simulink model "adc_preproc_core"  (R2012b)
settings: Solver=VariableStepDiscrete  SolverMode=SingleTasking  StartTime=0.0  StopTime=40960  RelTol=1e-3
undefined symbols (not defined in the file or in its folder): A, B, fixpnt, PCIN, xlipgetpartsetting
libraries: xbsIndex_r4 x537, casper_library_sources x8, casper_library_misc x8, simulink x1
(part 6 of 9)

== system adc_preproc_core/adc_preproc_core/noise_gen0/noise5/wgn/u2n ==
  u : Inport
  Delay : xbsIndex_r4/Delay  rst=off  infoeditControl=Selection of Reset will increase slice count due to use of real FFs and instead of SRLs  en=off  latency=1  dbl_ovrd=off  reg_retiming=off  block_type=delay
  Delay1 : xbsIndex_r4/Delay  rst=off  infoeditControl=Selection of Reset will increase slice count due to use of real FFs and instead of SRLs  en=off  latency=1  dbl_ovrd=off  reg_retiming=off  block_type=delay
  Delay2 : xbsIndex_r4/Delay  rst=off  infoeditControl=Selection of Reset will increase slice count due to use of real FFs and instead of SRLs  en=off  latency=1  dbl_ovrd=off  reg_retiming=off  block_type=delay
  Gateway Out : xbsIndex_r4/Gateway Out  inherit_from_input=off  hdl_port=off  timing_constraint=None  locs_specified=off  LOCs={}  UseAsDAC=off  DACChannel='1'  block_type=gatewayout
      settings: infoedit="Gateway out block.  Converts Xilinx fixed point inputs into ouputs of type Simulink integer, double, or fixed point.<P><P>Hardware notes:  In hardware these blocks become top level output ports or are discarded, depending on how they are configured."  xl_area=[0 0 0 0 17 0 0]  block_version=10.1.3
  Gateway Out1 : xbsIndex_r4/Gateway Out  inherit_from_input=off  hdl_port=off  timing_constraint=None  locs_specified=off  LOCs={}  UseAsDAC=off  DACChannel='1'  block_type=gatewayout
      settings: infoedit="Gateway out block.  Converts Xilinx fixed point inputs into ouputs of type Simulink integer, double, or fixed point.<P><P>Hardware notes:  In hardware these blocks become top level output ports or are discarded, depending on how they are configured."  xl_area=[0 0 0 0 17 0 0]  block_version=10.1.3
  Scope : Scope  NumInputPorts=2
      settings: YMin=-5~-5  YMax=5~5
  bottom_11 : xbsIndex_r4/Slice  nbits=11  boolean_output=off  mode=Lower Bit Location + Width  bit1=0  base1=MSB of Input  bit0=0  base0=LSB of Input  dbl_ovrd=off  block_type=slice
      settings: infoedit="Extracts a given range of bits from each input sample and presents it at the output.  The output type is ordinarily unsigned with binary point at zero, but can be Boolean when the slice is one bit wide.<P><P>Hardware notes: In hardware this block costs nothing."  block_version=10.1.3
  cosin_vanilla : Subsystem  AncestorBlock=casper_library_downconverter/cosin_vanilla  mask(cosin){output0=sin, output1=cos, phase=0, fraction=0, table_bits=11, n_bits=8, bin_pt=7, bram_latency=3, bram=BRAM, misc=off}
      mask prompts: output0 "first output function"; output1 "second output function"; phase "initial phase offset (?*(2*pi))"; fraction "fraction of cycle period to output (1/2^?)"; table_bits "samples in cycle period fraction to output (2^?)"; n_bits "bit width"; bin_pt "binary point"; bram_latency "bram latency"; bram "BRAM implementation"; misc "Miscellaneous port"
      mask init: same as adc_preproc_core/adc_preproc_core/noise_gen0/noise0/wgn/u2n/cosin_vanilla
      mask TypeOptions output0: sin | cos | -sin | -cos
      mask TypeOptions output1: none | sin | cos | -sin | -cos
      mask TypeOptions bram: distributed RAM | BRAM
      mask Display:
      | if ~(table_bits == 0),
      |         color('black');port_label('output',1,output0);
      |     color('black');port_label('output',2,output1);
      |     color('black');disp(['z^{-',num2str(bram_latency),'}'],'texmode','on');color('black');port_label('input',1,'theta');
      |     if strcmp(misc, 'on'),
      |         color('black');port_label('input',2,'misci');
      |         color('black');port_label('output',3,'misco');
      |     end
      | end
  log_lut : xbsIndex_r4/ROM  depth=2^11  initVector=fixpnt(sqrt(-2*log(linspace(2^-11,1,2^11))),9,7)  distributed_mem=Block RAM  rst=off  init_reg=0  en=off  latency=3  gui_display_data_type=Fixed-point  arith_type=Unsigned  n_bits=9  bin_pt=7  preci_type=Single  exp_width=8  frac_width=24  dbl_ovrd=off  optimize=Speed  use_rpm=off  block_type=sprom
      settings: xl_area=[0 0 1 0 0 0 0]  block_version=10.1.3
  r_cos : xbsIndex_r4/Mult  precision=Full  arith_type="Signed  (2's comp)"  n_bits=8  bin_pt=2  quantization=Truncate  overflow=Wrap  en=off  latency=3  dbl_ovrd=off  use_behavioral_HDL=off  opt=Speed  use_embedded=on  optimum_pipeline=off  pipeline=on  use_rpm=on  placement_style=Rectangular shape  block_type=mult
      settings: infoedit=Hardware notes: To use the internal pipeline stage of the dedicated multiplier you must select 'Pipeline for maximum performance'.  xl_area=[18 34 0 17 0 1 0]  block_version=10.1.3
  r_sin : xbsIndex_r4/Mult  precision=Full  arith_type="Signed  (2's comp)"  n_bits=8  bin_pt=2  quantization=Truncate  overflow=Wrap  en=off  latency=3  dbl_ovrd=off  use_behavioral_HDL=off  opt=Speed  use_embedded=on  optimum_pipeline=off  pipeline=on  use_rpm=on  placement_style=Rectangular shape  block_type=mult
      settings: infoedit=Hardware notes: To use the internal pipeline stage of the dedicated multiplier you must select 'Pipeline for maximum performance'.  xl_area=[18 34 0 17 0 1 0]  block_version=10.1.3
  top_11 : xbsIndex_r4/Slice  nbits=11  boolean_output=off  mode=Upper Bit Location + Width  bit1=0  base1=MSB of Input  bit0=0  base0=MSB of Input  dbl_ovrd=off  block_type=slice
      settings: infoedit="Extracts a given range of bits from each input sample and presents it at the output.  The output type is ordinarily unsigned with binary point at zero, but can be Boolean when the slice is one bit wide.<P><P>Hardware notes: In hardware this block costs nothing."  block_version=10.1.3
  n1 : Outport
  n2 : Outport  Port=2
  wires:
  Delay2/1 -> r_cos/2
  Delay1/1 -> r_sin/2
  Delay/1 -> r_sin/1, r_cos/1
  Gateway Out/1 -> Scope/1
  Gateway Out1/1 -> Scope/2
  bottom_11/1 -> cosin_vanilla/1(theta)
  top_11/1 -> log_lut/1
  u/1 -> top_11/1, bottom_11/1
  cosin_vanilla/2(cos) -> Delay2/1
  log_lut/1 -> Delay/1
  cosin_vanilla/1(sin) -> Delay1/1
  r_sin/1 -> Gateway Out/1, n1/1
  r_cos/1 -> Gateway Out1/1, n2/1

== system adc_preproc_core/adc_preproc_core/noise_gen0/noise6/wgn/u2n ==
  u : Inport
  Delay : xbsIndex_r4/Delay  rst=off  infoeditControl=Selection of Reset will increase slice count due to use of real FFs and instead of SRLs  en=off  latency=1  dbl_ovrd=off  reg_retiming=off  block_type=delay
  Delay1 : xbsIndex_r4/Delay  rst=off  infoeditControl=Selection of Reset will increase slice count due to use of real FFs and instead of SRLs  en=off  latency=1  dbl_ovrd=off  reg_retiming=off  block_type=delay
  Delay2 : xbsIndex_r4/Delay  rst=off  infoeditControl=Selection of Reset will increase slice count due to use of real FFs and instead of SRLs  en=off  latency=1  dbl_ovrd=off  reg_retiming=off  block_type=delay
  Gateway Out : xbsIndex_r4/Gateway Out  inherit_from_input=off  hdl_port=off  timing_constraint=None  locs_specified=off  LOCs={}  UseAsDAC=off  DACChannel='1'  block_type=gatewayout
      settings: infoedit="Gateway out block.  Converts Xilinx fixed point inputs into ouputs of type Simulink integer, double, or fixed point.<P><P>Hardware notes:  In hardware these blocks become top level output ports or are discarded, depending on how they are configured."  xl_area=[0 0 0 0 17 0 0]  block_version=10.1.3
  Gateway Out1 : xbsIndex_r4/Gateway Out  inherit_from_input=off  hdl_port=off  timing_constraint=None  locs_specified=off  LOCs={}  UseAsDAC=off  DACChannel='1'  block_type=gatewayout
      settings: infoedit="Gateway out block.  Converts Xilinx fixed point inputs into ouputs of type Simulink integer, double, or fixed point.<P><P>Hardware notes:  In hardware these blocks become top level output ports or are discarded, depending on how they are configured."  xl_area=[0 0 0 0 17 0 0]  block_version=10.1.3
  Scope : Scope  NumInputPorts=2
      settings: YMin=-5~-5  YMax=5~5
  bottom_11 : xbsIndex_r4/Slice  nbits=11  boolean_output=off  mode=Lower Bit Location + Width  bit1=0  base1=MSB of Input  bit0=0  base0=LSB of Input  dbl_ovrd=off  block_type=slice
      settings: infoedit="Extracts a given range of bits from each input sample and presents it at the output.  The output type is ordinarily unsigned with binary point at zero, but can be Boolean when the slice is one bit wide.<P><P>Hardware notes: In hardware this block costs nothing."  block_version=10.1.3
  cosin_vanilla : Subsystem  AncestorBlock=casper_library_downconverter/cosin_vanilla  mask(cosin){output0=sin, output1=cos, phase=0, fraction=0, table_bits=11, n_bits=8, bin_pt=7, bram_latency=3, bram=BRAM, misc=off}
      mask prompts: output0 "first output function"; output1 "second output function"; phase "initial phase offset (?*(2*pi))"; fraction "fraction of cycle period to output (1/2^?)"; table_bits "samples in cycle period fraction to output (2^?)"; n_bits "bit width"; bin_pt "binary point"; bram_latency "bram latency"; bram "BRAM implementation"; misc "Miscellaneous port"
      mask init: same as adc_preproc_core/adc_preproc_core/noise_gen0/noise0/wgn/u2n/cosin_vanilla
      mask TypeOptions output0: sin | cos | -sin | -cos
      mask TypeOptions output1: none | sin | cos | -sin | -cos
      mask TypeOptions bram: distributed RAM | BRAM
      mask Display:
      | if ~(table_bits == 0),
      |         color('black');port_label('output',1,output0);
      |     color('black');port_label('output',2,output1);
      |     color('black');disp(['z^{-',num2str(bram_latency),'}'],'texmode','on');color('black');port_label('input',1,'theta');
      |     if strcmp(misc, 'on'),
      |         color('black');port_label('input',2,'misci');
      |         color('black');port_label('output',3,'misco');
      |     end
      | end
  log_lut : xbsIndex_r4/ROM  depth=2^11  initVector=fixpnt(sqrt(-2*log(linspace(2^-11,1,2^11))),9,7)  distributed_mem=Block RAM  rst=off  init_reg=0  en=off  latency=3  gui_display_data_type=Fixed-point  arith_type=Unsigned  n_bits=9  bin_pt=7  preci_type=Single  exp_width=8  frac_width=24  dbl_ovrd=off  optimize=Speed  use_rpm=off  block_type=sprom
      settings: xl_area=[0 0 1 0 0 0 0]  block_version=10.1.3
  r_cos : xbsIndex_r4/Mult  precision=Full  arith_type="Signed  (2's comp)"  n_bits=8  bin_pt=2  quantization=Truncate  overflow=Wrap  en=off  latency=3  dbl_ovrd=off  use_behavioral_HDL=off  opt=Speed  use_embedded=on  optimum_pipeline=off  pipeline=on  use_rpm=on  placement_style=Rectangular shape  block_type=mult
      settings: infoedit=Hardware notes: To use the internal pipeline stage of the dedicated multiplier you must select 'Pipeline for maximum performance'.  xl_area=[18 34 0 17 0 1 0]  block_version=10.1.3
  r_sin : xbsIndex_r4/Mult  precision=Full  arith_type="Signed  (2's comp)"  n_bits=8  bin_pt=2  quantization=Truncate  overflow=Wrap  en=off  latency=3  dbl_ovrd=off  use_behavioral_HDL=off  opt=Speed  use_embedded=on  optimum_pipeline=off  pipeline=on  use_rpm=on  placement_style=Rectangular shape  block_type=mult
      settings: infoedit=Hardware notes: To use the internal pipeline stage of the dedicated multiplier you must select 'Pipeline for maximum performance'.  xl_area=[18 34 0 17 0 1 0]  block_version=10.1.3
  top_11 : xbsIndex_r4/Slice  nbits=11  boolean_output=off  mode=Upper Bit Location + Width  bit1=0  base1=MSB of Input  bit0=0  base0=MSB of Input  dbl_ovrd=off  block_type=slice
      settings: infoedit="Extracts a given range of bits from each input sample and presents it at the output.  The output type is ordinarily unsigned with binary point at zero, but can be Boolean when the slice is one bit wide.<P><P>Hardware notes: In hardware this block costs nothing."  block_version=10.1.3
  n1 : Outport
  n2 : Outport  Port=2
  wires:
  Delay2/1 -> r_cos/2
  Delay1/1 -> r_sin/2
  Delay/1 -> r_sin/1, r_cos/1
  Gateway Out/1 -> Scope/1
  Gateway Out1/1 -> Scope/2
  bottom_11/1 -> cosin_vanilla/1(theta)
  top_11/1 -> log_lut/1
  u/1 -> top_11/1, bottom_11/1
  cosin_vanilla/2(cos) -> Delay2/1
  log_lut/1 -> Delay/1
  cosin_vanilla/1(sin) -> Delay1/1
  r_sin/1 -> Gateway Out/1, n1/1
  r_cos/1 -> Gateway Out1/1, n2/1

== system adc_preproc_core/adc_preproc_core/noise_gen0/noise7/wgn/u2n ==
  u : Inport
  Delay : xbsIndex_r4/Delay  rst=off  infoeditControl=Selection of Reset will increase slice count due to use of real FFs and instead of SRLs  en=off  latency=1  dbl_ovrd=off  reg_retiming=off  block_type=delay
  Delay1 : xbsIndex_r4/Delay  rst=off  infoeditControl=Selection of Reset will increase slice count due to use of real FFs and instead of SRLs  en=off  latency=1  dbl_ovrd=off  reg_retiming=off  block_type=delay
  Delay2 : xbsIndex_r4/Delay  rst=off  infoeditControl=Selection of Reset will increase slice count due to use of real FFs and instead of SRLs  en=off  latency=1  dbl_ovrd=off  reg_retiming=off  block_type=delay
  Gateway Out : xbsIndex_r4/Gateway Out  inherit_from_input=off  hdl_port=off  timing_constraint=None  locs_specified=off  LOCs={}  UseAsDAC=off  DACChannel='1'  block_type=gatewayout
      settings: infoedit="Gateway out block.  Converts Xilinx fixed point inputs into ouputs of type Simulink integer, double, or fixed point.<P><P>Hardware notes:  In hardware these blocks become top level output ports or are discarded, depending on how they are configured."  xl_area=[0 0 0 0 17 0 0]  block_version=10.1.3
  Gateway Out1 : xbsIndex_r4/Gateway Out  inherit_from_input=off  hdl_port=off  timing_constraint=None  locs_specified=off  LOCs={}  UseAsDAC=off  DACChannel='1'  block_type=gatewayout
      settings: infoedit="Gateway out block.  Converts Xilinx fixed point inputs into ouputs of type Simulink integer, double, or fixed point.<P><P>Hardware notes:  In hardware these blocks become top level output ports or are discarded, depending on how they are configured."  xl_area=[0 0 0 0 17 0 0]  block_version=10.1.3
  Scope : Scope  NumInputPorts=2
      settings: YMin=-5~-5  YMax=5~5
  bottom_11 : xbsIndex_r4/Slice  nbits=11  boolean_output=off  mode=Lower Bit Location + Width  bit1=0  base1=MSB of Input  bit0=0  base0=LSB of Input  dbl_ovrd=off  block_type=slice
      settings: infoedit="Extracts a given range of bits from each input sample and presents it at the output.  The output type is ordinarily unsigned with binary point at zero, but can be Boolean when the slice is one bit wide.<P><P>Hardware notes: In hardware this block costs nothing."  block_version=10.1.3
  cosin_vanilla : Subsystem  AncestorBlock=casper_library_downconverter/cosin_vanilla  mask(cosin){output0=sin, output1=cos, phase=0, fraction=0, table_bits=11, n_bits=8, bin_pt=7, bram_latency=3, bram=BRAM, misc=off}
      mask prompts: output0 "first output function"; output1 "second output function"; phase "initial phase offset (?*(2*pi))"; fraction "fraction of cycle period to output (1/2^?)"; table_bits "samples in cycle period fraction to output (2^?)"; n_bits "bit width"; bin_pt "binary point"; bram_latency "bram latency"; bram "BRAM implementation"; misc "Miscellaneous port"
      mask init: same as adc_preproc_core/adc_preproc_core/noise_gen0/noise0/wgn/u2n/cosin_vanilla
      mask TypeOptions output0: sin | cos | -sin | -cos
      mask TypeOptions output1: none | sin | cos | -sin | -cos
      mask TypeOptions bram: distributed RAM | BRAM
      mask Display:
      | if ~(table_bits == 0),
      |         color('black');port_label('output',1,output0);
      |     color('black');port_label('output',2,output1);
      |     color('black');disp(['z^{-',num2str(bram_latency),'}'],'texmode','on');color('black');port_label('input',1,'theta');
      |     if strcmp(misc, 'on'),
      |         color('black');port_label('input',2,'misci');
      |         color('black');port_label('output',3,'misco');
      |     end
      | end
  log_lut : xbsIndex_r4/ROM  depth=2^11  initVector=fixpnt(sqrt(-2*log(linspace(2^-11,1,2^11))),9,7)  distributed_mem=Block RAM  rst=off  init_reg=0  en=off  latency=3  gui_display_data_type=Fixed-point  arith_type=Unsigned  n_bits=9  bin_pt=7  preci_type=Single  exp_width=8  frac_width=24  dbl_ovrd=off  optimize=Speed  use_rpm=off  block_type=sprom
      settings: xl_area=[0 0 1 0 0 0 0]  block_version=10.1.3
  r_cos : xbsIndex_r4/Mult  precision=Full  arith_type="Signed  (2's comp)"  n_bits=8  bin_pt=2  quantization=Truncate  overflow=Wrap  en=off  latency=3  dbl_ovrd=off  use_behavioral_HDL=off  opt=Speed  use_embedded=on  optimum_pipeline=off  pipeline=on  use_rpm=on  placement_style=Rectangular shape  block_type=mult
      settings: infoedit=Hardware notes: To use the internal pipeline stage of the dedicated multiplier you must select 'Pipeline for maximum performance'.  xl_area=[18 34 0 17 0 1 0]  block_version=10.1.3
  r_sin : xbsIndex_r4/Mult  precision=Full  arith_type="Signed  (2's comp)"  n_bits=8  bin_pt=2  quantization=Truncate  overflow=Wrap  en=off  latency=3  dbl_ovrd=off  use_behavioral_HDL=off  opt=Speed  use_embedded=on  optimum_pipeline=off  pipeline=on  use_rpm=on  placement_style=Rectangular shape  block_type=mult
      settings: infoedit=Hardware notes: To use the internal pipeline stage of the dedicated multiplier you must select 'Pipeline for maximum performance'.  xl_area=[18 34 0 17 0 1 0]  block_version=10.1.3
  top_11 : xbsIndex_r4/Slice  nbits=11  boolean_output=off  mode=Upper Bit Location + Width  bit1=0  base1=MSB of Input  bit0=0  base0=MSB of Input  dbl_ovrd=off  block_type=slice
      settings: infoedit="Extracts a given range of bits from each input sample and presents it at the output.  The output type is ordinarily unsigned with binary point at zero, but can be Boolean when the slice is one bit wide.<P><P>Hardware notes: In hardware this block costs nothing."  block_version=10.1.3
  n1 : Outport
  n2 : Outport  Port=2
  wires:
  r_cos/1 -> n2/1, Gateway Out1/1
  r_sin/1 -> n1/1, Gateway Out/1
  cosin_vanilla/1(sin) -> Delay1/1
  log_lut/1 -> Delay/1
  cosin_vanilla/2(cos) -> Delay2/1
  u/1 -> bottom_11/1, top_11/1
  top_11/1 -> log_lut/1
  bottom_11/1 -> cosin_vanilla/1(theta)
  Gateway Out1/1 -> Scope/2
  Gateway Out/1 -> Scope/1
  Delay/1 -> r_cos/1, r_sin/1
  Delay1/1 -> r_sin/2
  Delay2/1 -> r_cos/2

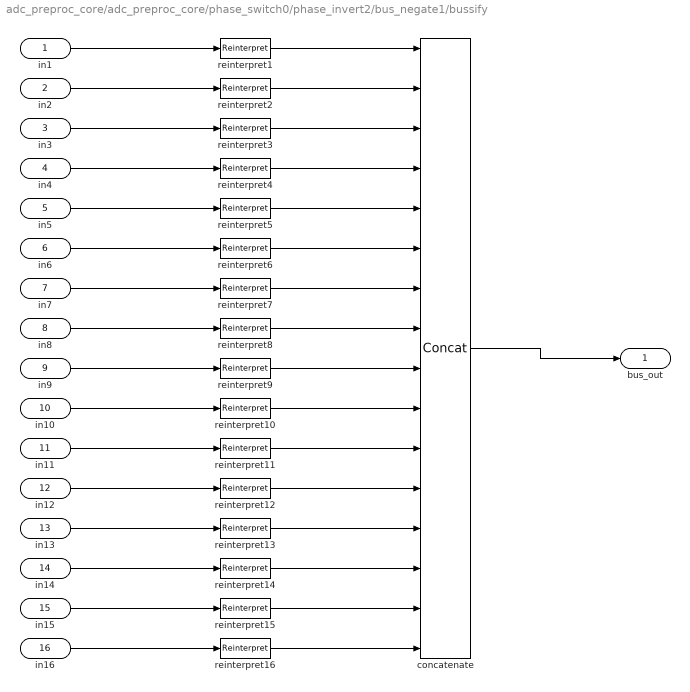
== system adc_preproc_core/adc_preproc_core/phase_switch0/phase_invert2/bus_negate1/bussify ==
  in1 : Inport
  in2 : Inport  Port=2
  in3 : Inport  Port=3
  in4 : Inport  Port=4
  in5 : Inport  Port=5
  in6 : Inport  Port=6
  in7 : Inport  Port=7
  in8 : Inport  Port=8
  in9 : Inport  Port=9
  in10 : Inport  Port=10
  in11 : Inport  Port=11
  in12 : Inport  Port=12
  in13 : Inport  Port=13
  in14 : Inport  Port=14
  in15 : Inport  Port=15
  in16 : Inport  Port=16
  concatenate : xbsIndex_r4/Concat  num_inputs=16  dbl_ovrd=off  block_type=concat
  reinterpret{1..16} (16 alike) : xbsIndex_r4/Reinterpret  force_arith_type=on  arith_type=Unsigned  force_bin_pt=on  bin_pt=0  block_type=reinterpret
      reinterpret1 settings: infoedit="Changes signal type without altering the binary representation.   You can changed the signal between signed and unsigned, and relocate the binary point.<br><br>Hardware notes: In hardware this block costs nothing.<br><br>Example:  Suppose the input is 6 bits wide, signed, with 2 fractional bits, and the output is forced to unsigned with 0 fractional bits.  Then an input of -2.0 (1110.00 in binary 2's complement) becomes an output of 56 (111000 in binary)."
  bus_out : Outport
  wires:
  reinterpret16/1 -> concatenate/16
  in16/1 -> reinterpret16/1
  reinterpret15/1 -> concatenate/15
  in15/1 -> reinterpret15/1
  reinterpret14/1 -> concatenate/14
  in14/1 -> reinterpret14/1
  reinterpret13/1 -> concatenate/13
  in13/1 -> reinterpret13/1
  reinterpret12/1 -> concatenate/12
  in12/1 -> reinterpret12/1
  reinterpret11/1 -> concatenate/11
  in11/1 -> reinterpret11/1
  reinterpret10/1 -> concatenate/10
  in10/1 -> reinterpret10/1
  reinterpret9/1 -> concatenate/9
  in9/1 -> reinterpret9/1
  reinterpret8/1 -> concatenate/8
  in8/1 -> reinterpret8/1
  reinterpret7/1 -> concatenate/7
  in7/1 -> reinterpret7/1
  reinterpret6/1 -> concatenate/6
  in6/1 -> reinterpret6/1
  reinterpret5/1 -> concatenate/5
  in5/1 -> reinterpret5/1
  reinterpret4/1 -> concatenate/4
  in4/1 -> reinterpret4/1
  reinterpret3/1 -> concatenate/3
  in3/1 -> reinterpret3/1
  reinterpret2/1 -> concatenate/2
  in2/1 -> reinterpret2/1
  reinterpret1/1 -> concatenate/1
  in1/1 -> reinterpret1/1
  concatenate/1 -> bus_out/1

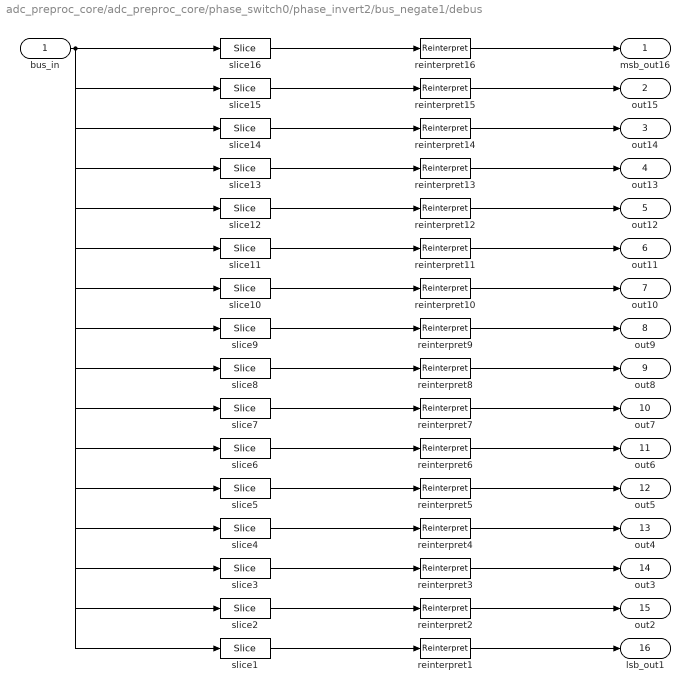
== system adc_preproc_core/adc_preproc_core/phase_switch0/phase_invert2/bus_negate1/debus ==
  bus_in : Inport
  reinterpret{1..16} (16 alike) : xbsIndex_r4/Reinterpret  force_arith_type=on  arith_type="Signed  (2's comp)"  force_bin_pt=on  bin_pt=7  block_type=reinterpret
  slice1 : xbsIndex_r4/Slice  nbits=8  boolean_output=off  mode=Upper Bit Location + Width  bit1=-120  base1=MSB of Input  bit0=0  base0=LSB of Input  dbl_ovrd=off  block_type=slice
  slice10 : xbsIndex_r4/Slice  nbits=8  boolean_output=off  mode=Upper Bit Location + Width  bit1=-48  base1=MSB of Input  bit0=0  base0=LSB of Input  dbl_ovrd=off  block_type=slice
  slice11 : xbsIndex_r4/Slice  nbits=8  boolean_output=off  mode=Upper Bit Location + Width  bit1=-40  base1=MSB of Input  bit0=0  base0=LSB of Input  dbl_ovrd=off  block_type=slice
  slice12 : xbsIndex_r4/Slice  nbits=8  boolean_output=off  mode=Upper Bit Location + Width  bit1=-32  base1=MSB of Input  bit0=0  base0=LSB of Input  dbl_ovrd=off  block_type=slice
  slice13 : xbsIndex_r4/Slice  nbits=8  boolean_output=off  mode=Upper Bit Location + Width  bit1=-24  base1=MSB of Input  bit0=0  base0=LSB of Input  dbl_ovrd=off  block_type=slice
  slice14 : xbsIndex_r4/Slice  nbits=8  boolean_output=off  mode=Upper Bit Location + Width  bit1=-16  base1=MSB of Input  bit0=0  base0=LSB of Input  dbl_ovrd=off  block_type=slice
  slice15 : xbsIndex_r4/Slice  nbits=8  boolean_output=off  mode=Upper Bit Location + Width  bit1=-8  base1=MSB of Input  bit0=0  base0=LSB of Input  dbl_ovrd=off  block_type=slice
  slice16 : xbsIndex_r4/Slice  nbits=8  boolean_output=off  mode=Upper Bit Location + Width  bit1=0  base1=MSB of Input  bit0=0  base0=LSB of Input  dbl_ovrd=off  block_type=slice
  slice2 : xbsIndex_r4/Slice  nbits=8  boolean_output=off  mode=Upper Bit Location + Width  bit1=-112  base1=MSB of Input  bit0=0  base0=LSB of Input  dbl_ovrd=off  block_type=slice
  slice3 : xbsIndex_r4/Slice  nbits=8  boolean_output=off  mode=Upper Bit Location + Width  bit1=-104  base1=MSB of Input  bit0=0  base0=LSB of Input  dbl_ovrd=off  block_type=slice
  slice4 : xbsIndex_r4/Slice  nbits=8  boolean_output=off  mode=Upper Bit Location + Width  bit1=-96  base1=MSB of Input  bit0=0  base0=LSB of Input  dbl_ovrd=off  block_type=slice
  slice5 : xbsIndex_r4/Slice  nbits=8  boolean_output=off  mode=Upper Bit Location + Width  bit1=-88  base1=MSB of Input  bit0=0  base0=LSB of Input  dbl_ovrd=off  block_type=slice
  slice6 : xbsIndex_r4/Slice  nbits=8  boolean_output=off  mode=Upper Bit Location + Width  bit1=-80  base1=MSB of Input  bit0=0  base0=LSB of Input  dbl_ovrd=off  block_type=slice
  slice7 : xbsIndex_r4/Slice  nbits=8  boolean_output=off  mode=Upper Bit Location + Width  bit1=-72  base1=MSB of Input  bit0=0  base0=LSB of Input  dbl_ovrd=off  block_type=slice
  slice8 : xbsIndex_r4/Slice  nbits=8  boolean_output=off  mode=Upper Bit Location + Width  bit1=-64  base1=MSB of Input  bit0=0  base0=LSB of Input  dbl_ovrd=off  block_type=slice
  slice9 : xbsIndex_r4/Slice  nbits=8  boolean_output=off  mode=Upper Bit Location + Width  bit1=-56  base1=MSB of Input  bit0=0  base0=LSB of Input  dbl_ovrd=off  block_type=slice
  msb_out16 : Outport
  out15 : Outport  Port=2
  out14 : Outport  Port=3
  out13 : Outport  Port=4
  out12 : Outport  Port=5
  out11 : Outport  Port=6
  out10 : Outport  Port=7
  out9 : Outport  Port=8
  out8 : Outport  Port=9
  out7 : Outport  Port=10
  out6 : Outport  Port=11
  out5 : Outport  Port=12
  out4 : Outport  Port=13
  out3 : Outport  Port=14
  out2 : Outport  Port=15
  lsb_out1 : Outport  Port=16
  wires:
  bus_in/1 -> slice16/1, slice15/1, slice14/1, slice13/1, slice12/1, slice11/1, slice10/1, slice9/1, slice8/1, slice7/1, slice6/1, slice5/1, slice4/1, slice3/1, slice2/1, slice1/1
  slice16/1 -> reinterpret16/1
  reinterpret16/1 -> msb_out16/1
  slice15/1 -> reinterpret15/1
  reinterpret15/1 -> out15/1
  slice14/1 -> reinterpret14/1
  reinterpret14/1 -> out14/1
  slice13/1 -> reinterpret13/1
  reinterpret13/1 -> out13/1
  slice12/1 -> reinterpret12/1
  reinterpret12/1 -> out12/1
  slice11/1 -> reinterpret11/1
  reinterpret11/1 -> out11/1
  slice10/1 -> reinterpret10/1
  reinterpret10/1 -> out10/1
  slice9/1 -> reinterpret9/1
  reinterpret9/1 -> out9/1
  slice8/1 -> reinterpret8/1
  reinterpret8/1 -> out8/1
  slice7/1 -> reinterpret7/1
  reinterpret7/1 -> out7/1
  slice6/1 -> reinterpret6/1
  reinterpret6/1 -> out6/1
  slice5/1 -> reinterpret5/1
  reinterpret5/1 -> out5/1
  slice4/1 -> reinterpret4/1
  reinterpret4/1 -> out4/1
  slice3/1 -> reinterpret3/1
  reinterpret3/1 -> out3/1
  slice2/1 -> reinterpret2/1
  reinterpret2/1 -> out2/1
  slice1/1 -> reinterpret1/1
  reinterpret1/1 -> lsb_out1/1

== system adc_preproc_core/adc_preproc_core/noise_gen0/noise0/wgn/u2n/cosin_vanilla ==
  theta : Inport
  Delay : xbsIndex_r4/Delay  rst=off  infoeditControl=Selection of Reset will increase slice count due to use of real FFs and instead of SRLs  en=off  latency=bram_latency  dbl_ovrd=off  reg_retiming=on  block_type=delay
  ROM : xbsIndex_r4/ROM  depth=2^(11)  initVector=[127 127 383 383 639 639 639 895 895 1151 1151 1151 1407 1407 1407 1663 1663 1919 1919 1919 2175 2175 2431 2431 2431 2687 2687 2943 2943 2943 3199 3199 3455 3455 3455 3711 3711 3711 3967 3967 4223 4223 4223 4479 4479 4735 4735 4735 4991 4991 5246 5246 5246 5502 5502 5502 5758 5758 6014 6014 6014 6270 6270 6526 6526 6525 6781 6781 7037 7037 7037 7293 7293 7293 7549 7549 7805 7804 7804 8060 8060 8060 8316 8316 8572 8572 8572 8827 8827 9083 9083 9083 9339 9339 9339 9595 9594 9850 9850 9850 10106 10106 10106 10362 10362 10617 10617 10617 10873 10873 10873 11129 11129 11128 11384 11384 11640 11640 11640 11896 11895 11895 12151 12151 12407 12407 12407 12662 12662 12662 12918 12918 12918 13173 13173 13429 13429 13429 13685 13685 13684 13940 13940 13940 14196 14196 14195 14451 14451 14451 14707 14707 14962 14962 14962 15218 15218 15217 15473 15473 15473 15729 15729 15728 15984 15984 15984 16240 16239 16239 16495 16495 16495 16750 16750 16750 17006 17006 17005 17261 17261 17261 17517 17516 17516 17772 17772 17772 18027 18027 18027 18283 18282 18282 18538 18538 18538 18793 18793 18793 19049 19048 19048 19304 19304 19304 19559 19559 19559 19815 19814 19814 20070 20070 20069 20069 20325 20325 20324 20580 20580 20580 20835 20835 20835 21091 21090 21090 21090 21346 21345 21345 21601 21601 21600 21600 21856 21856 21855 22111 22111 22111 22366 22366 22366 22366 22621 22621 22621 22876 22876 22876 22876 23131 23131 23131 23387 23386 23386 23386 23641 23641 23641 23641 23896 23896 23896 24151 24151 24151 24151 24406 24406 24406 24405 24661 24661 24660 24660 24916 24916 24915 24915 25171 25170 25170 25170 25426 25425 25425 25425 25680 25680 25680 25679 25935 25935 25934 25934 26190 26190 26189 26189 26445 26444 26444 26444 26699 26699 26699 26698 26698 26954 26953 26953 26953 27208 27208 27208 27207 27207 27463 27462 27462 27462 27717 27717 27717 27716 27716 27972 27971 27971 27971 27970 28226 28226 28225 28225 28225 28480 28480 28480 28479 28479 28735 28734 28734 28734 28733 28989 28989 28988 28988 28988 28987 29243 29243 29242 29242 29242 29497 29497 29496 29496 29496 29495 29751 29751 29750 29750 29750 29749 30005 30005 30004 30004 30004 30003 30003 30258 30258 30258 30257 30257 30257 30512 30512 30512 30511 30511 30510 30510 30766 30765 30765 30765 30764 30764 30763 31019 31019 31018 31018 31018 31017 31017 31017 31272 31272 31271 31271 31271 31270 31270 31270 31269 31525 31524 31524 31524 31523 31523 31523 31522 31522 31777 31777 31777 31776 31776 31775 31775 31775 31774 31774 32030 32029 32029 32028 32028 32028 32027 32027 32027 32026 32026 32025 32281 32281 32280 32280 32279 32279 32279 32278 32278 32277 32277 32277 32276 32276 32276 32531 32531 32530 32530 32530 32529 32529 32528 32528 32528 32527 32527 32526 32526 32526 32525 32525 32525 32524 32524 32523 32523 32523 32522 32522 32521 32521 32521 32520 32520 32519 32519 32519 32518 32518 32517 32517 32517 32516 32516 32516 32515 32515 32514 32514 32514 32513 32513 32512 32512 32512 32767 32767 32766 32766 32766 32765 32765 32764 32764 32764 32763 32763 32763 32762 32762 32761 32761 32761 32760 32760 32759 32759 32759 32758 32758 32757 32757 32757 32756 32756 32755 32755 32755 32754 32754 32754 32753 32753 32752 32752 32752 32751 32751 32750 32750 32750 32749 32749 32492 32492 32492 32491 32491 32491 32490 32490 32489 32489 32489 32488 32488 32487 32487 32231 32230 32230 32229 32229 32229 32228 32228 32228 32227 32227 32226 31970 31970 31969 31969 31969 31968 31968 31967 31967 31967 31710 31710 31709 31709 31709 31708 31708 31708 31707 31451 31450 31450 31450 31449 31449 31449 31448 31448 31191 31191 31191 31190 31190 31190 31189 31189 30933 30932 30932 30931 30931 30931 30930 30674 30674 30673 30673 30672 30672 30672 30415 30415 30415 30414 30414 30414 30157 30157 30156 30156 30156 30155 30155 29899 29898 29898 29898 29897 29897 29641 29640 29640 29640 29639 29639 29382 29382 29382 29381 29381 29125 29124 29124 29124 29123 29123 28867 28866 28866 28866 28865 28609 28609 28608 28608 ...(+8071 chars)]  distributed_mem=Block RAM  rst=off  init_reg=0  en=off  latency=bram_latency  gui_display_data_type=Fixed-point  arith_type=Unsigned  n_bits=n_bits*2  bin_pt=0  preci_type=Single  exp_width=8  frac_width=24  dbl_ovrd=off  optimize=Speed  use_rpm=on  block_type=sprom
  assert : xbsIndex_r4/Assert  assert_type=on  type_source=Explicitly  gui_display_data_type=Fixed-point  arith_type=Unsigned  n_bits=11  bin_pt=0  preci_type=Single  exp_width=8  frac_width=24  assert_rate=off  rate_source=Explicitly  period=1  output_port=on  block_type=assert
  c_to_ri : casper_library_misc/c_to_ri  n_bits=n_bits  bin_pt=bin_pt
      settings: AttributesFormatString=8_7 r/i
  misci : xbsIndex_r4/Constant  const=0  gui_display_data_type=Fixed-point  arith_type=Unsigned  n_bits=1  bin_pt=0  preci_type=Single  exp_width=8  frac_width=24  explicit_period=on  period=1  equ=P=C  opselect=C  inp2=PCIN>>17  opr=+  inp1=P  carry=CIN  dbl_ovrd=off  block_type=constant
  misco : Terminator
  sin : Outport
  cos : Outport  Port=2
  wires:
  Delay/1 -> misco/1
  misci/1 -> Delay/1
  c_to_ri/2 -> cos/1
  c_to_ri/1 -> sin/1
  ROM/1 -> c_to_ri/1
  assert/1 -> ROM/1
  theta/1 -> assert/1
